simulink model "systemmain_dynblock"  (R2017b)
settings: Solver=VariableStepAuto  StartTime=0.0  StopTime=10  RelTol=1e-3
settings Model: Creator=DanAdmin  LastModifiedBy=DanAdmin

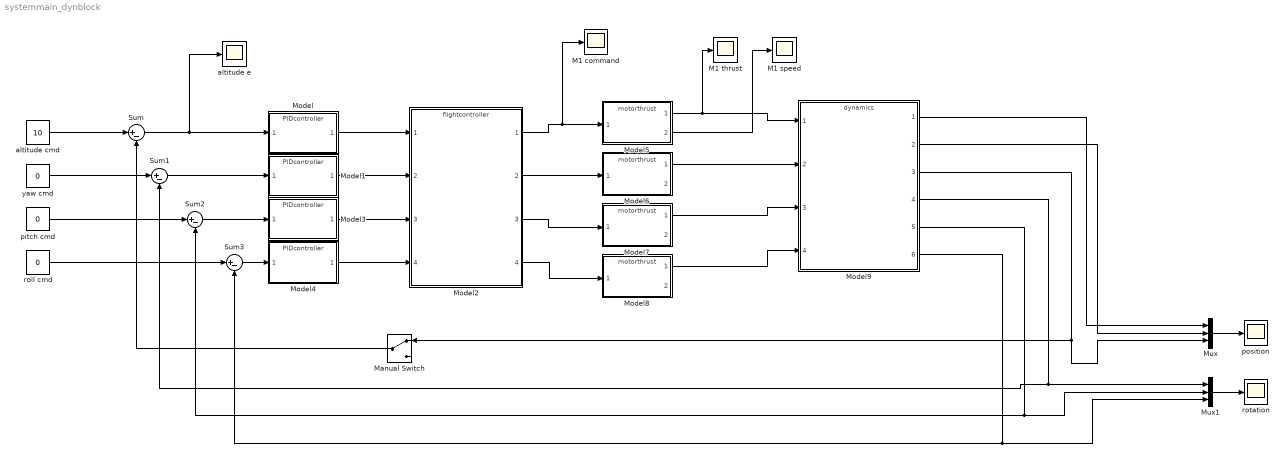
== system systemmain_dynblock ==
  M1 command : Scope
  M1 speed : Scope
  M1 thrust : Scope
  Manual Switch : ManualSwitch
  Model{,1,3..4} (4 alike) : ModelReference  ModelNameDialog=PIDcontroller.slx  SimulationMode=Normal  ModelReferenceVersion=1.10
  Model2 : ModelReference  ModelNameDialog=flightcontroller.slx  SimulationMode=Normal  ModelReferenceVersion=1.10
  Model{5..8} (4 alike) : ModelReference  ModelNameDialog=motorthrust.slx  SimulationMode=Normal  ModelReferenceVersion=1.20
  Model9 : ModelReference  ModelNameDialog=dynamics.slx  SimulationMode=Normal  ModelReferenceVersion=1.15
  Mux : Mux  Inputs=3
  Mux1 : Mux  Inputs=3
  Sum{,1..3} (4 alike) : Sum  Inputs=|+-
  altitude cmd : Constant  Value=10
  altitude e : Scope
  pitch cmd : Constant  Value=0
  "position " : Scope
  roll cmd : Constant  Value=0
  rotation : Scope
  yaw cmd : Constant  Value=0
  wires:
  Model4/1 -> Model2/4
  Model/1 -> Model2/1
  Model3/1 -> Model2/3
  Model1/1 -> Model2/2
  Model2/1 -> M1 command/1, Model5/1
  Model2/2 -> Model6/1
  Model2/3 -> Model7/1
  Model2/4 -> Model8/1
  Sum/1 -> altitude e/1, Model/1
  Sum3/1 -> Model4/1
  Sum2/1 -> Model3/1
  Sum1/1 -> Model1/1
  Model9/4 -> Sum1/2, Mux1/1
  Model9/5 -> Mux1/2, Sum2/2
  Model9/6 -> Mux1/3, Sum3/2
  Model9/3 -> Mux/3, Manual Switch/1
  roll cmd/1 -> Sum3/1
  pitch cmd/1 -> Sum2/1
  yaw cmd/1 -> Sum1/1
  altitude cmd/1 -> Sum/1
  Mux1/1 -> rotation/1
  Mux/1 -> "position "/1
  Model9/1 -> Mux/1
  Model9/2 -> Mux/2
  Model5/1 -> M1 thrust/1, Model9/1
  Model6/1 -> Model9/2
  Model7/1 -> Model9/3
  Model8/1 -> Model9/4
  Model5/2 -> M1 speed/1
  Manual Switch/1 -> Sum/2
